simulink model "dynInv"  (R2020a)
settings: Solver=VariableStepAuto  StartTime=0.0  StopTime=20  RelTol=1e-3
values from neighbouring files (symbols this model uses):
  Along = [Xu Xa 0 -g ... (first row only)    [b747_LQR_PID.m]
  Blong = [Xde;Zde/U1;Mde+(Madot*Zde)/U1;0]    [b747_LQR_PID.m]
  CA = Clong_alpha*Along    [b747_LQR_PID.m]
  CBinv = inv(Clong_alpha*Blong)    [b747_LQR_PID.m]
  Clong = eye(length(Along))    [b747_LQR_PID.m]
  Clong_alpha = [0 1 0 0]    [b747_LQR_PID.m]
  Dlong = zeros(size(Clong,1),size(Blong,2))    [b747_LQR_PID.m]
  k = 5    [b747_LQR_PID.m]
libraries: simulink_extras x6
settings Model: Creator=aaron  LastModifiedBy=aaron

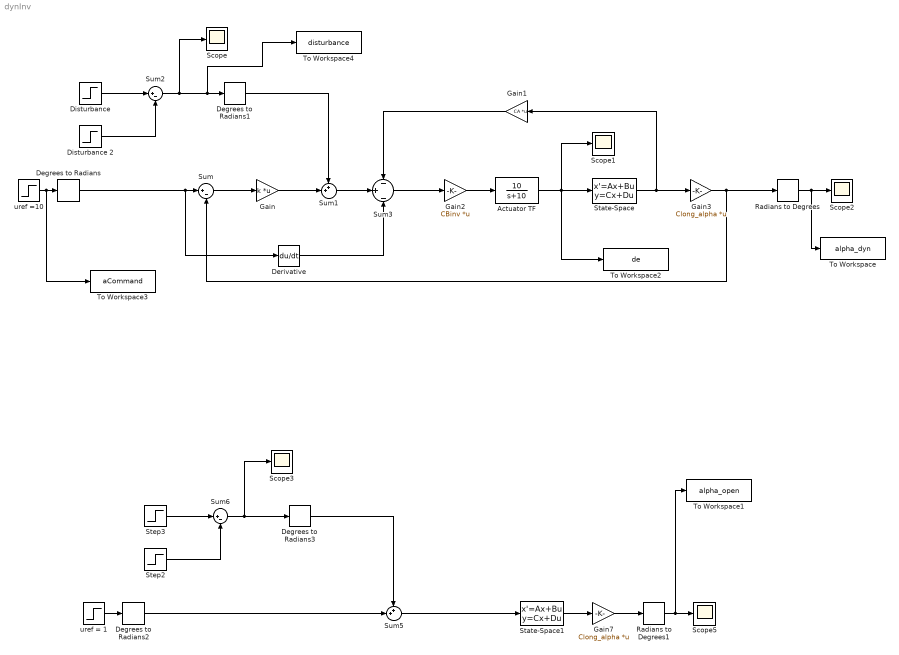
== system dynInv ==
  Actuator TF : TransferFcn  Numerator=[10]  Denominator=[1 10]
  Degrees to Radians{,1..3} (4 alike) : simulink_extras/Transformations/Degrees to Radians
  Derivative : Derivative
  Disturbance : Step  After=15  SampleTime=0
  Disturbance 2 : Step  Time=3  After=15  SampleTime=0
  Gain : Gain  Gain=k  Multiplication=Matrix(K*u)
  Gain1 : Gain  Gain=CA  Multiplication=Matrix(K*u)
  Gain2 : Gain  Gain=CBinv  Multiplication=Matrix(K*u)
  Gain3 : Gain  Gain=Clong_alpha  Multiplication=Matrix(K*u)
  Gain7 : Gain  Gain=Clong_alpha  Multiplication=Matrix(K*u)
  Radians to Degrees : simulink_extras/Transformations/Radians to Degrees
  Radians to Degrees1 : simulink_extras/Transformations/Radians to Degrees
  Scope{,1..3,5} (5 alike) : Scope
  State-Space : StateSpace  A=Along  B=Blong  C=Clong  D=Dlong  InitialCondition=0
  State-Space1 : StateSpace  A=Along  B=Blong  C=Clong  D=Dlong  InitialCondition=0
  Step2 : Step  Time=3  After=45  SampleTime=0
  Step3 : Step  After=45  SampleTime=0
  Sum : Sum  Inputs=|+-
  Sum1 : Sum  Inputs=++|
  Sum2 : Sum  Inputs=|+-
  Sum3 : Sum  Inputs=-|+|-
  Sum5 : Sum  Inputs=++|
  Sum6 : Sum  Inputs=|+-
  To Workspace : ToWorkspace  VariableName=alpha_dyn  SampleTime=-1
  To Workspace1 : ToWorkspace  VariableName=alpha_open  SampleTime=-1
  To Workspace2 : ToWorkspace  VariableName=de  SampleTime=-1
  To Workspace3 : ToWorkspace  VariableName=aCommand  SampleTime=-1
  To Workspace4 : ToWorkspace  VariableName=disturbance  SampleTime=-1
  uref = 1 : Step  After=10  SampleTime=0
  uref =10 : Step  After=10  SampleTime=0
  wires:
  Sum/1 -> Gain/1
  Gain/1 -> Sum1/2
  Sum2/1 -> Scope/1, To Workspace4/1, Degrees to Radians1/1
  uref =10/1 -> To Workspace3/1, Degrees to Radians/1
  Sum1/1 -> Sum3/2
  Gain1/1 -> Sum3/1
  Sum3/1 -> Gain2/1
  Gain2/1 -> Actuator TF/1
  Actuator TF/1 -> To Workspace2/1, State-Space/1, Scope1/1
  Radians to Degrees/1 -> To Workspace/1, Scope2/1
  Gain3/1 -> Radians to Degrees/1, Sum/2
  Derivative/1 -> Sum3/3
  State-Space/1 -> Gain3/1, Gain1/1
  Degrees to Radians/1 -> Derivative/1, Sum/1
  Disturbance/1 -> Sum2/1
  Disturbance 2/1 -> Sum2/2
  Degrees to Radians1/1 -> Sum1/1
  Sum5/1 -> State-Space1/1
  Gain7/1 -> Radians to Degrees1/1
  Radians to Degrees1/1 -> To Workspace1/1, Scope5/1
  State-Space1/1 -> Gain7/1
  Sum6/1 -> Scope3/1, Degrees to Radians3/1
  Step2/1 -> Sum6/2
  uref = 1/1 -> Degrees to Radians2/1
  Step3/1 -> Sum6/1
  Degrees to Radians3/1 -> Sum5/1
  Degrees to Radians2/1 -> Sum5/2
